simulink model "se_pll_reduced_order_runtime"  (R2026a)
settings: Solver=ode45  StopTime=2.0  MaxStep=1e-3
undefined symbols (not defined in the file or in its folder): activePowerBias, activePowerScales, disturbanceAmplitude, modalFrequency, responseGain, sagDropGain, zeta
settings Model: Creator=yao  LastModifiedBy=yao

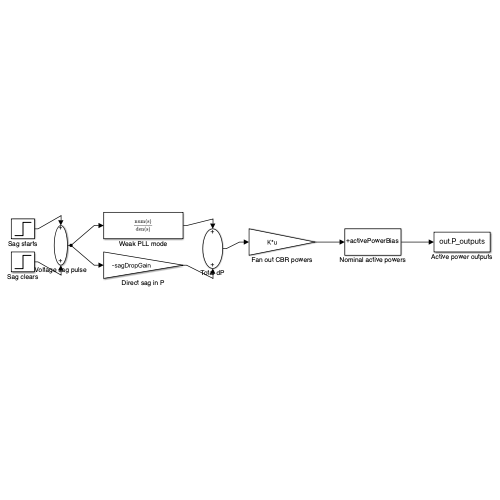
[thumbnail: Simulink's stored preview of the top-level diagram]
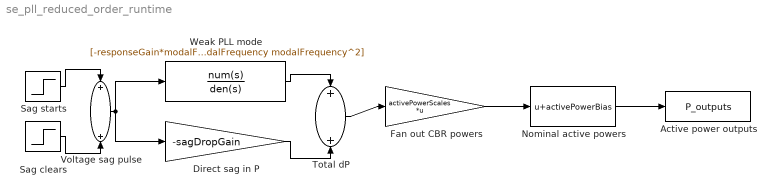
== system se_pll_reduced_order_runtime ==
  Active power outputs : ToWorkspace  VariableName=P_outputs  SaveFormat=Timeseries  SampleTime=-1
  Direct sag in P : Gain  Gain=-sagDropGain
  Fan out CBR powers : Gain  Gain=activePowerScales  Multiplication=Matrix(K*u)
  Nominal active powers : Bias  Bias=activePowerBias  SaturateOnIntegerOverflow=off
  Sag clears : Step  Time=0.12  FinalValue=-disturbanceAmplitude  SampleTime=0
  Sag starts : Step  Time=0.10  FinalValue=disturbanceAmplitude  SampleTime=0
  Total dP : Sum
  Voltage sag pulse : Sum
  Weak PLL mode : TransferFcn  Numerator=[-responseGain*modalFrequency^2 0]  Denominator=[1 2*zeta*modalFrequency modalFrequency^2]
  wires:
  Sag starts/1 -> Voltage sag pulse/1
  Sag clears/1 -> Voltage sag pulse/2
  Voltage sag pulse/1 -> Weak PLL mode/1, Direct sag in P/1
  Weak PLL mode/1 -> Total dP/1
  Direct sag in P/1 -> Total dP/2
  Total dP/1 -> Fan out CBR powers/1
  Fan out CBR powers/1 -> Nominal active powers/1
  Nominal active powers/1 -> Active power outputs/1
